simulink model "chap17_6sim"  (Simulink 7.7)
settings: Solver=ode45  StartTime=0.0  StopTime=10  RelTol=1e-5
settings Model: Creator=ljk  LastModifiedBy=ljk  ExtModeTrigMode=oneshot  ExtModeArmWhenConnect=off
settings DataIOCC: LimitDataPoints=off  SignalLoggingName=sigsOut
settings OptimizationCC: BooleanDataType=off  InitFltsAndDblsToZero=on
settings DebuggingCC: SaveWithParameterizedLinksMsg=none  SignalResolutionControl=TryResolveAllWithWarning  SolverPrmCheckMsg=none  MultiTaskDSMMsg=warning  MultiTaskCondExecSysMsg=none  StrictBusMsg=None
settings HardwareCC: TargetUnknown=on
settings RTWCC: IncludeERTFirstTime=on
settings GRTTargetCC: TargetFcnLib=ansi_tfl_tmw.mat

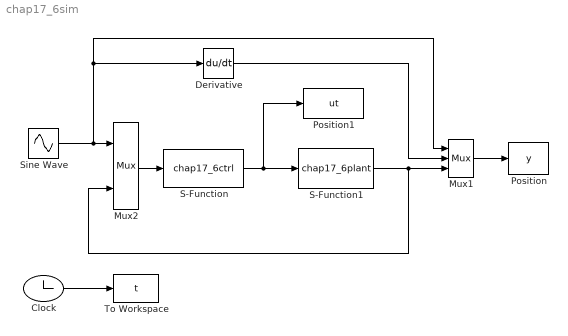
== system chap17_6sim ==
  Clock : Clock
      settings: Decimation=10
  Derivative : Derivative
  Mux1 : Mux  Inputs=3
  Mux2 : Mux  Inputs=2
  Position : ToWorkspace  VariableName=y  SampleTime=-1  SaveFormat=Array
  Position1 : ToWorkspace  VariableName=ut  SampleTime=-1  SaveFormat=Array
  S-Function : S-Function  FunctionName=chap17_6ctrl  EnableBusSupport=off
  S-Function1 : S-Function  FunctionName=chap17_6plant  EnableBusSupport=off
  Sine Wave : Sin  Amplitude=0.1  SampleTime=0
  To Workspace : ToWorkspace  VariableName=t  SampleTime=-1  SaveFormat=Array
  wires:
  Mux1/1 -> Position/1
  S-Function1/1 -> Mux2/2, Mux1/3
  S-Function/1 -> S-Function1/1, Position1/1
  Clock/1 -> To Workspace/1
  Sine Wave/1 -> Mux2/1, Mux1/1, Derivative/1
  Mux2/1 -> S-Function/1
  Derivative/1 -> Mux1/2
